simulink subsystem "mouvementtranslation"  (R2023a)
settings: Solver=VariableStepAuto  StartTime=0.0  StopTime=10.0  RelTol=1e-3
undefined symbols (not defined in the file or in its folder): g
settings Model: Creator=raphb  LastModifiedBy=raphb

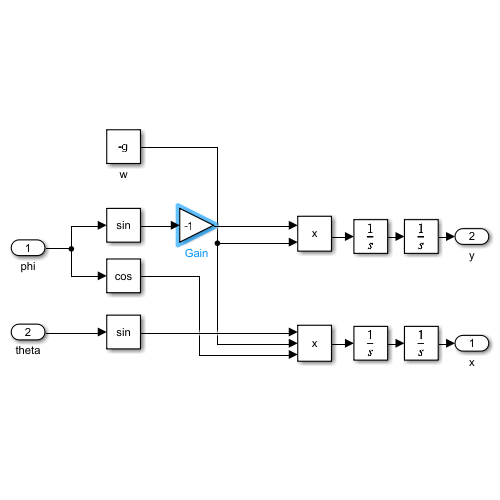
[thumbnail: Simulink's stored preview of the top-level diagram]
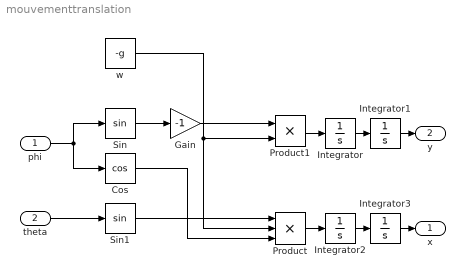
== system mouvementtranslation ==
  phi : Inport
  theta : Inport  Port=2
  Cos : Trigonometry  Operator=cos
  Gain : Gain  Gain=-1
  Integrator{,1..3} (4 alike) : Integrator
  Product : Product  Inputs=3
  Product1 : Product
  Sin : Trigonometry
  Sin1 : Trigonometry
  w : Constant  Value=-g
  x : Outport
  y : Outport  Port=2
  wires:
  phi/1 -> Cos/1, Sin/1
  theta/1 -> Sin1/1
  Sin1/1 -> Product/1
  w/1 -> Product/2, Product1/2
  Cos/1 -> Product/3
  Integrator1/1 -> y/1
  Product1/1 -> Integrator/1
  Integrator/1 -> Integrator1/1
  Product/1 -> Integrator2/1
  Integrator2/1 -> Integrator3/1
  Integrator3/1 -> x/1
  Sin/1 -> Gain/1
  Gain/1 -> Product1/1
